simulink model "event_triggered_vs_pid"  (R2026a)
settings: Solver=ode4  StopTime=20.0  FixedStep=0.001  MaxStep=0.001
libraries: slpidlib x1

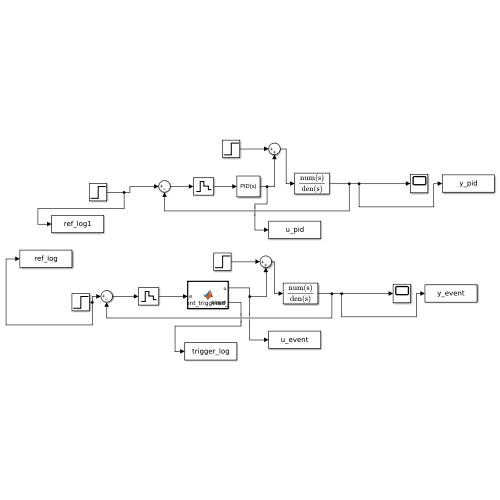
[thumbnail: Simulink's stored preview of the top-level diagram]
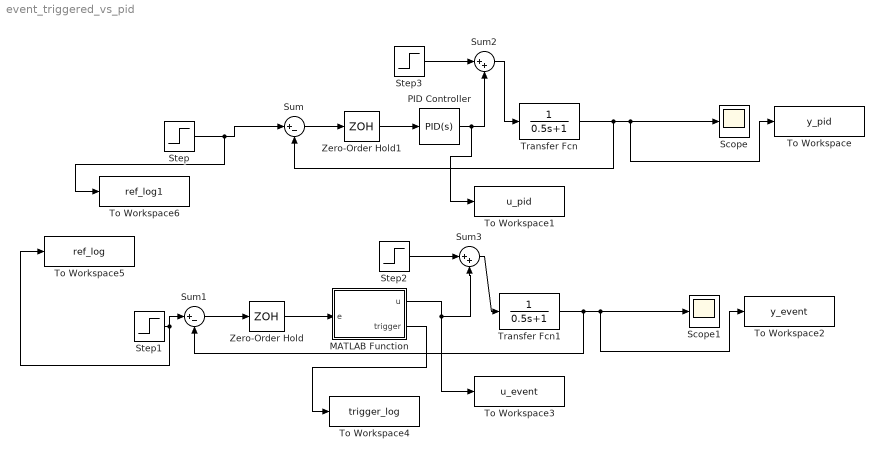
== system event_triggered_vs_pid ==
  MATLAB Function : MATLAB Function  TreatAsAtomicUnit=on
  PID Controller : slpidlib/PID Controller  Controller=PID  Form=Parallel  TimeDomain=Continuous-time  UseExternalTs=off  SampleTime=-1  IntegratorMethod=Forward Euler  FilterMethod=Forward Euler  ControllerParametersSource=internal  P=2  I=5  UseKiTs=off  D=0.1  UseExternalDerivativeSource=off  N=100  UseFilter=on  TunerSelectOption=Transfer Function Based (PID Tuner App)  InitialConditionSource=internal  InitialConditionForIntegrator=0  InitialConditionForFilter=0  DifferentiatorICPrevScaledInput=0  ExternalReset=none  TrackingMode=off  Kt=1  LimitOutput=off  SatLimitsSource=internal  UpperSaturationLimit=inf  LowerSaturationLimit=-inf  LinearizeAsGain=on  AntiWindupMode=none  Kb=1  LimitIntegrator=off  UpperIntegratorSaturationLimit=inf  LowerIntegratorSaturationLimit=-inf  POutMin=[]  POutMax=[]  IOutMin=[]  IOutMax=[]  DOutMin=[]  DOutMax=[]  NOutMin=[]  NOutMax=[]  SumOutMin=[]  SumOutMax=[]  SaturationOutMin=[]  SaturationOutMax=[]  PParamMin=[]  PParamMax=[]  IParamMin=[]  IParamMax=[]  DParamMin=[]  DParamMax=[]  NParamMin=[]  NParamMax=[]  KbParamMin=[]  KbParamMax=[]  KtParamMin=[]  KtParamMax=[]  KbOutMin=[]  KbOutMax=[]  KtOutMin=[]  KtOutMax=[]  IntegratorOutMin=[]  IntegratorOutMax=[]  FilterOutMin=[]  FilterOutMax=[]  SumI1OutMin=[]  SumI1OutMax=[]  SumI2OutMin=[]  SumI2OutMax=[]  SumI3OutMin=[]  SumI3OutMax=[]  SumI4OutMin=[]  SumI4OutMax=[]  SumDOutMin=[]  SumDOutMax=[]  DifferentiatorOutMin=[]  DifferentiatorOutMax=[]  FilterDiffOutCoefMin=[]  FilterDiffOutCoefMax=[]  ReciprocalOutMin=[]  ReciprocalOutMax=[]  SumDenOutMin=[]  SumDenOutMax=[]  SumNumOutMin=[]  SumNumOutMax=[]  DivideOutMin=[]  DivideOutMax=[]  UdiffTsProdOutMin=[]  UdiffTsProdOutMax=[]  NTsProdOutMin=[]  NTsProdOutMax=[]  UintegralTsProdOutMin=[]  UintegralTsProdOutMax=[]  UngainTsProdOutMin=[]  UngainTsProdOutMax=[]  ClampingZeroOutDataTypeStr=Inherit: Inherit via back propagation  ClampingZeroOutMin=[]  ClampingZeroOutMax=[]  FilterDenConstantOutDataTypeStr=Inherit: Inherit via back propagation  FilterDenConstantOutMin=[]  FilterDenConstantOutMax=[]  PCopyOutDataTypeStr=Inherit: Inherit via back propagation  PCopyOutMin=[]  PCopyOutMax=[]  NCopyOutDataTypeStr=Inherit: Inherit via back propagation  NCopyOutMin=[]  NCopyOutMax=[]  IntegratorContinuousStateAttributes=''  IntegratorStateMustResolveToSignalObject=off  IntegratorRTWStateStorageClass=Auto  FilterContinuousStateAttributes=''  FilterStateMustResolveToSignalObject=off  FilterRTWStateStorageClass=Auto  ParallelPVariant=InternalParameters  IdealPVariant=Disabled  IVariant=InternalParameters  DVariant=InternalParameters  IntegratorVariant=Continuous  SatVariant=Disabled  AWVariant=Passthrough  PCopyVariant=Disabled  TRVariant=Disabled  FdbkBlocksVariant=Forward  IdealPFdbkVariant=Disabled  SatFdbkVariant=Disabled  DerivativeFilterVariant=ContFilter  NVariant=InternalParameters  NCopyVariant=Disabled  FilterICVariant=InternalICsFilter  IntegratorICVariant=InternalICs  ExternalResetVariant=Disabled  TRSumVariant=Passthrough  SumFdbkVariant=Disabled  SumVariant=Sum_PID  TsampFilterVariant=InternalTs  TsampNgainVariant=Passthrough  TsampIntegralVariant=Disabled_SignalSpec  ExternalSaturationOutDataTypeStr=Inherit: Same as second input  DerivativeSourceVariant=ErrorSignal  PreIntVariant=InternalPreInt
  Scope : Scope
  Scope1 : Scope
  Step : Step  Time=2  FinalValue=10  SampleTime=0
  Step1 : Step  Time=2  FinalValue=10  SampleTime=0
  Step2 : Step  Time=10  SampleTime=0
  Step3 : Step  Time=10  SampleTime=0
  Sum : Sum  Inputs=|+-
  Sum1 : Sum  Inputs=|+-
  Sum2 : Sum  Inputs=|++
  Sum3 : Sum  Inputs=|++
  To Workspace : ToWorkspace  VariableName=y_pid  SampleTime=-1
  To Workspace1 : ToWorkspace  VariableName=u_pid  SampleTime=-1
  To Workspace2 : ToWorkspace  VariableName=y_event  SampleTime=-1
  To Workspace3 : ToWorkspace  VariableName=u_event  SampleTime=-1
  To Workspace4 : ToWorkspace  VariableName=trigger_log  SampleTime=-1
  To Workspace5 : ToWorkspace  VariableName=ref_log  SampleTime=-1
  To Workspace6 : ToWorkspace  VariableName=ref_log1  SampleTime=-1
  Transfer Fcn : TransferFcn  Denominator=[0.5 1]
  Transfer Fcn1 : TransferFcn  Denominator=[0.5 1]
  Zero-Order Hold : ZeroOrderHold  SampleTime=0.001
  Zero-Order Hold1 : ZeroOrderHold  SampleTime=0.02
  wires:
  Sum/1 -> Zero-Order Hold1/1
  PID Controller/1 -> Sum2/2, To Workspace1/1
  Transfer Fcn/1 -> To Workspace/1, Scope/1, Sum/2
  Step/1 -> To Workspace6/1, Sum/1
  Sum1/1 -> Zero-Order Hold/1
  Step1/1 -> Sum1/1, To Workspace5/1
  Transfer Fcn1/1 -> To Workspace2/1, Scope1/1, Sum1/2
  MATLAB Function/1(u) -> Sum3/2, To Workspace3/1
  MATLAB Function/2(trigger) -> To Workspace4/1
  Step2/1 -> Sum3/1
  Step3/1 -> Sum2/1
  Sum3/1 -> Transfer Fcn1/1
  Sum2/1 -> Transfer Fcn/1
  Zero-Order Hold/1 -> MATLAB Function/1(e)
  Zero-Order Hold1/1 -> PID Controller/1

== matlab function event_triggered_vs_pid/MATLAB Function ==
  data: e input; u output; trigger output
function [u, trigger] = event_triggered_pid(e)
    persistent e_last u_hold integral_term prev_e counter
    if isempty(e_last)
        e_last = 0; u_hold = 0; integral_term = 0; prev_e = 0; counter = 0;
    end

    Kp = 2; Ki = 5; Kd = 0.1;
    threshold = 0.05;
    dt = 0.001;
    max_hold_steps = 500;   % force an update at least every 0.5s

    integral_term = integral_term + e*dt;   % always accumulate — this is cheap
    derivative_term = (e - prev_e)/dt;
    prev_e = e;
    counter = counter + 1;

    if abs(e - e_last) >= threshold || counter >= max_hold_steps
        u_hold = Kp*e + Ki*integral_term + Kd*derivative_term;
        e_last = e;
        counter = 0;
        trigger = 1;
    else
        trigger = 0;
    end
    u = u_hold;
end
